simulink model "Even_odd"  (R2024b)
settings: Solver=VariableStepAuto  StartTime=0.0  StopTime=inf  RelTol=1e-3
settings Model: Creator=rohan  LastModifiedBy=rohan

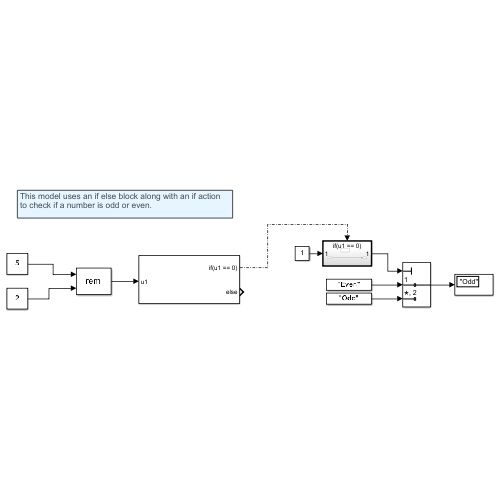
[thumbnail: Simulink's stored preview of the top-level diagram]
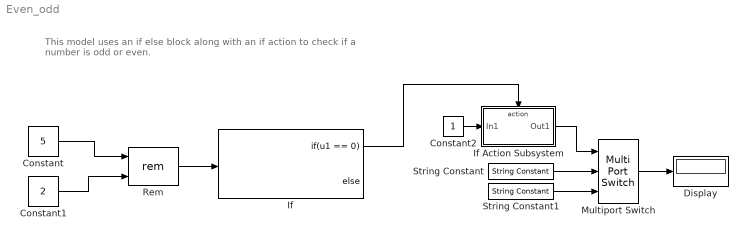
== system Even_odd ==
  note: This model uses an if else block along with an if action
      | to check if a number is odd or even.
  Constant : Constant  Value=5
  Constant1 : Constant  Value=2
  Constant2 : Constant
  Display : Display
  If : If  IfExpression=u1 == 0
  If Action Subsystem : Subsystem  TreatAsAtomicUnit=on
  Multiport Switch : MultiPortSwitch  Inputs=2  DiagnosticForDefault=None  SaturateOnIntegerOverflow=off  InputSameDT=off
  Rem : Math  Operator=rem
  String Constant : StringConstant  String="\"Even\""
  String Constant1 : StringConstant  String="\"Odd\""
  wires:
  Constant/1 -> Rem/1
  Constant1/1 -> Rem/2
  Rem/1 -> If/1
  If/1 -> If Action Subsystem/Action
  If Action Subsystem/1(Out1) -> Multiport Switch/1
  Constant2/1 -> If Action Subsystem/1(In1)
  String Constant/1 -> Multiport Switch/2
  String Constant1/1 -> Multiport Switch/3
  Multiport Switch/1 -> Display/1

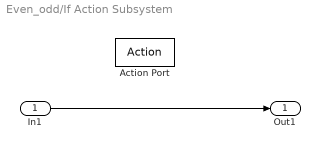
== system Even_odd/If Action Subsystem ==
  In1 : Inport
  Action Port : ActionPort  ActionPortLabel=if(u1 == 0)
  Out1 : Outport
  wires:
  In1/1 -> Out1/1
